simulink library "controller_cl"  (R2018a)
settings: Solver=VariableStepAuto  StartTime=0.0  StopTime=10.0  RelTol=1e-3
libraries: headingSetpointCalculation_cl x1
settings Model: Creator=mcobb  LastModifiedBy=mcobb

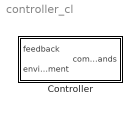
== system controller_cl ==
  Controller : Subsystem

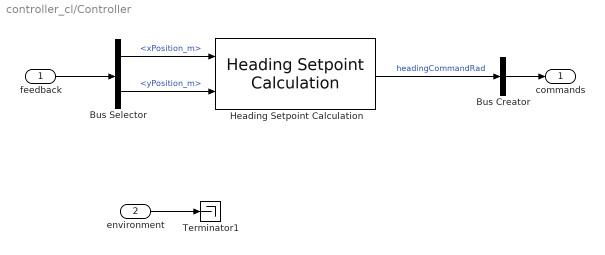
== system controller_cl/Controller ==
  feedback : Inport
  environment : Inport  Port=2
  Bus Creator : BusCreator  Inputs=1
  Bus Selector : BusSelector  OutputSignals=xPosition_m,yPosition_m
  Heading Setpoint Calculation : headingSetpointCalculation_cl/Heading Setpoint Calculation
  Terminator1 : Terminator
  commands : Outport
  wires:
  feedback/1 -> Bus Selector/1
  environment/1 -> Terminator1/1
  Heading Setpoint Calculation/1 -> Bus Creator/1  "headingCommandRad"
  Bus Creator/1 -> commands/1
  Bus Selector/1 -> Heading Setpoint Calculation/1  "<xPosition_m>"
  Bus Selector/2 -> Heading Setpoint Calculation/2  "<yPosition_m>"
